simulink model "Nonlinear_LQG_Robust_A"  (R2019b)
settings: Solver=VariableStepAuto  StartTime=0.0  StopTime=10  RelTol=1e-3
values from neighbouring files (symbols this model uses):
  b = 0.2    [HOMEWORK..m]
  g = 9.81    [HOMEWORK..m]
  K = lqr(A,B,Q,R)    [HOMEWORK..m]
  M = M_1*1.05+m    (= 11.3)    [HOMEWORK..m]
  m = 1.64    [HOMEWORK..m]
  Nu = NxNu(5)    [HOMEWORK..m]
  Nx = NxNu(1:4,:)    [HOMEWORK..m]
  sysKF = ss(A-K_kalman*C,[B K_kalman],eye(4),0*[B K_kalman])    [HOMEWORK..m]
  x0 = [x_0_1 x_0_2 x_0_3 x_0_4]'    [HOMEWORK..m]
  x_0_1 = -0.01    [HOMEWORK..m]
  x_0_2 = 0.01    [HOMEWORK..m]
  x_0_3 = 0.05    [HOMEWORK..m]
  x_0_4 = 0.1    [HOMEWORK..m]
undefined symbols (not defined in the file or in its folder): J, L
settings Model: Creator=Sina  LastModifiedBy=Harris
settings OptimizationCC: LifeSpan=inf
settings DebuggingCC: SFExecutionAtInitializationDiag=none  ArithmeticOperatorsInVariantConditions=warning
settings SFSimCC: CustomCodeUndefinedFunction=UseInterfaceOnly
settings CodeAppCC: StateflowObjectComments=on

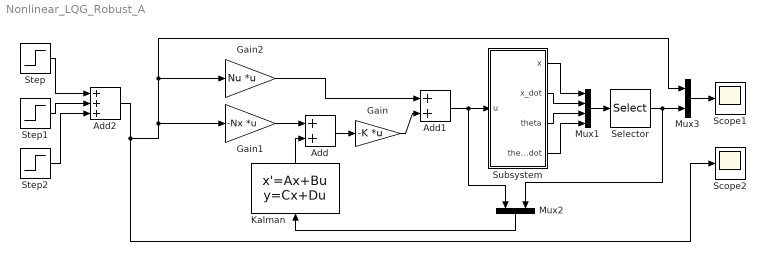
== system Nonlinear_LQG_Robust_A ==
  Add : Sum
  Add1 : Sum
  Add2 : Sum  Inputs=+++
  Gain : Gain  Gain=-K  Multiplication=Matrix(K*u)
  Gain1 : Gain  Gain=-Nx  Multiplication=Matrix(K*u)
  Gain2 : Gain  Gain=Nu  Multiplication=Matrix(K*u)
  Kalman : StateSpace  A=sysKF.a  B=sysKF.b  C=sysKF.c  D=sysKF.d  InitialCondition=x0
  Mux1 : Mux
  Mux2 : Mux  Inputs=2
  Mux3 : Mux  Inputs=2
  Scope1 : Scope
  Scope2 : Scope
  Selector : Selector  InputPortWidth=4  IndexOptions=Index vector (dialog)  Indices=1  OutputSizes=1
  Step : Step  Time=15  SampleTime=0
  Step1 : Step  Time=25  After=-2  SampleTime=0
  Step2 : Step  Time=35  SampleTime=0
  Subsystem : Subsystem
  wires:
  Gain1/1 -> Add/1
  Selector/1 -> Mux2/2, Mux3/2
  Mux1/1 -> Selector/1
  Mux2/1 -> Kalman/1
  Subsystem/4(theta_dot) -> Mux1/4
  Subsystem/1(x) -> Mux1/1
  Add1/1 -> Subsystem/1(u), Mux2/1
  Gain2/1 -> Add1/1
  Add/1 -> Gain/1
  Kalman/1 -> Add/2
  Subsystem/2(x_dot) -> Mux1/2
  Mux3/1 -> Scope1/1
  Step/1 -> Add2/1
  Add2/1 -> Gain1/1, Gain2/1, Mux3/1, Scope2/1
  Step2/1 -> Add2/3
  Step1/1 -> Add2/2
  Gain/1 -> Add1/2
  Subsystem/3(theta) -> Mux1/3

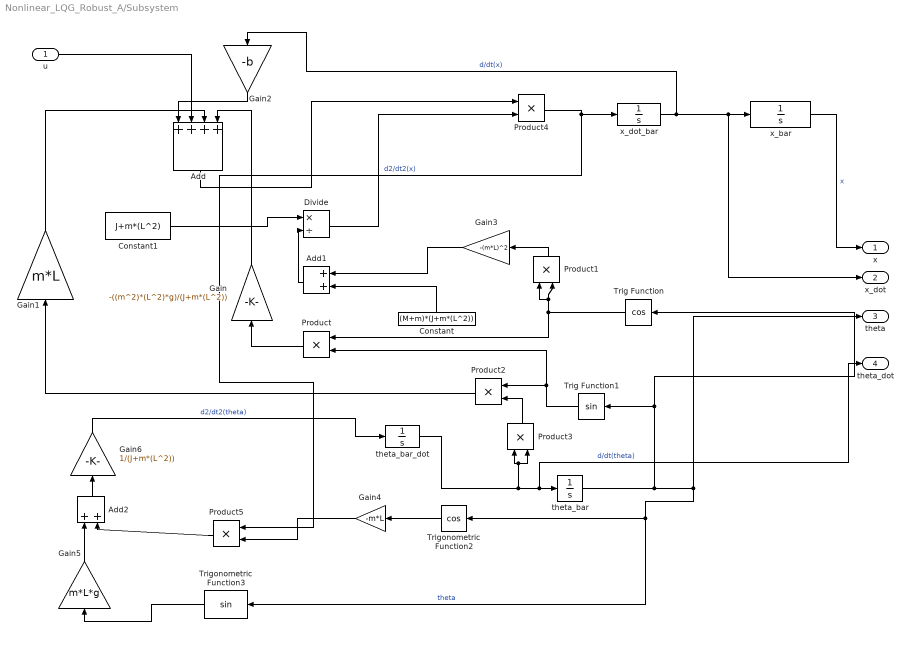
== system Nonlinear_LQG_Robust_A/Subsystem ==
  u : Inport
  Add : Sum  Inputs=++++
  Add1 : Sum
  Add2 : Sum
  Constant : Constant  Value=(M+m)*(J+m*(L^2))
  Constant1 : Constant  Value=J+m*(L^2)
  Divide : Product  Inputs=*/
  Gain : Gain  Gain=-((m^2)*(L^2)*g)/(J+m*(L^2))
  Gain1 : Gain  Gain=m*L
  Gain2 : Gain  Gain=-b
  Gain3 : Gain  Gain=-(m*L)^2
  Gain4 : Gain  Gain=-m*L
  Gain5 : Gain  Gain=m*L*g
  Gain6 : Gain  Gain=1/(J+m*(L^2))
  Product{,1..5} (6 alike) : Product
  Trig Function : Trigonometry  Operator=cos
  Trig Function1 : Trigonometry
  Trigonometric Function2 : Trigonometry  Operator=cos
  Trigonometric Function3 : Trigonometry
  theta_bar : Integrator  InitialCondition=x_0_3
  theta_bar_dot : Integrator  InitialCondition=x_0_4
  x_bar : Integrator  InitialCondition=x_0_1
  x_dot_bar : Integrator  InitialCondition=x_0_2
  x : Outport
  x_dot : Outport  Port=2
  theta : Outport  Port=3
  theta_dot : Outport  Port=4
  wires:
  x_dot_bar/1 -> x_dot/1, x_bar/1, Gain2/1  "d/dt(x)"
  Trig Function/1 -> Product/1, Product1/1, Product1/2
  Product4/1 -> Product5/1, x_dot_bar/1  "d2/dt2(x)"
  x_bar/1 -> x/1  "x"
  theta_bar_dot/1 -> theta_dot/1, theta_bar/1, Product3/1, Product3/2  "d/dt(theta)"
  theta_bar/1 -> theta/1, Trigonometric Function3/1, Trigonometric Function2/1, Trig Function/1, Trig Function1/1  "theta"
  Constant/1 -> Add1/2
  Trig Function1/1 -> Product/2, Product2/1
  Product5/1 -> Add2/2
  Product3/1 -> Product2/2
  Trigonometric Function2/1 -> Gain4/1
  Gain1/1 -> Add/3
  Product2/1 -> Gain1/1
  Product/1 -> Gain/1
  Gain2/1 -> Add/1
  Gain5/1 -> Add2/1
  Trigonometric Function3/1 -> Gain5/1
  Add1/1 -> Divide/2
  Gain4/1 -> Product5/2
  Add/1 -> Product4/1
  Divide/1 -> Product4/2
  Gain6/1 -> theta_bar_dot/1  "d2/dt2(theta)"
  Add2/1 -> Gain6/1
  Gain/1 -> Add/4
  Constant1/1 -> Divide/1
  u/1 -> Add/2
  Gain3/1 -> Add1/1
  Product1/1 -> Gain3/1
